simulink model "Deviation"  (R2021b)
settings: Solver=VariableStepAuto  StartTime=0.0  StopTime=100  RelTol=1e-3
undefined symbols (not defined in the file or in its folder): A, B, B_pseudoinverse, C, F, K
settings Model: Creator=Asus  LastModifiedBy=Asus

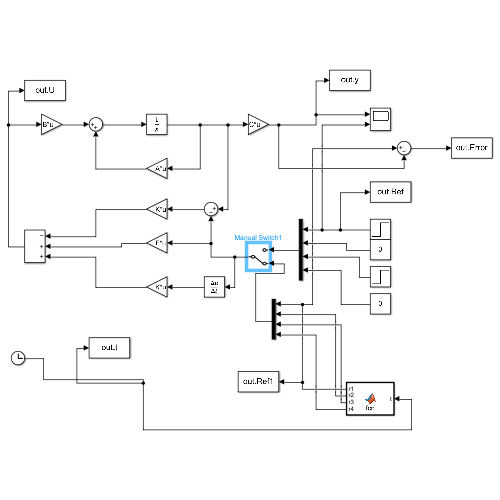
[thumbnail: Simulink's stored preview of the top-level diagram]
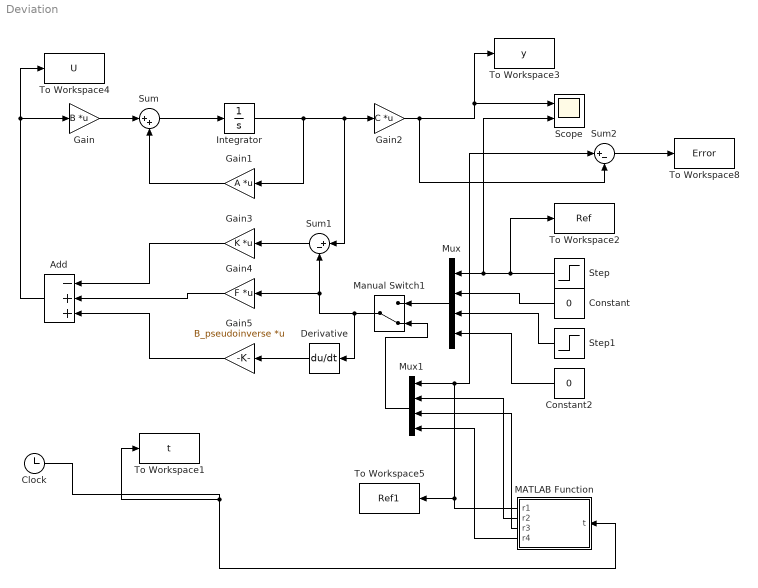
== system Deviation ==
  Add : Sum  Inputs=-++
  Clock : Clock
  Constant : Constant  Value=0
  Constant2 : Constant  Value=0
  Derivative : Derivative
  Gain : Gain  Gain=B  Multiplication=Matrix(K*u)
  Gain1 : Gain  Gain=A  Multiplication=Matrix(K*u)
  Gain2 : Gain  Gain=C  Multiplication=Matrix(K*u)
  Gain3 : Gain  Gain=K  Multiplication=Matrix(K*u)
  Gain4 : Gain  Gain=F  Multiplication=Matrix(K*u)
  Gain5 : Gain  Gain=B_pseudoinverse  Multiplication=Matrix(K*u)
  Integrator : Integrator
  MATLAB Function : MATLAB Function  TreatAsAtomicUnit=on
  Manual Switch1 : ManualSwitch  CurrentSetting=0
  Mux : Mux
  Mux1 : Mux
  Scope : Scope  NumInputPorts=2
  Step : Step  After=10  SampleTime=0
  Step1 : Step  After=10  SampleTime=0
  Sum : Sum  Inputs=|++
  Sum1 : Sum  Inputs=|+-
  Sum2 : Sum  Inputs=|+-
  To Workspace1 : ToWorkspace  VariableName=t  SaveFormat=Timeseries  SampleTime=-1
  To Workspace2 : ToWorkspace  VariableName=Ref  SaveFormat=Timeseries  SampleTime=-1
  To Workspace3 : ToWorkspace  VariableName=y  SaveFormat=Timeseries  SampleTime=-1
  To Workspace4 : ToWorkspace  VariableName=U  SaveFormat=Timeseries  SampleTime=-1
  To Workspace5 : ToWorkspace  VariableName=Ref1  SaveFormat=Timeseries  SampleTime=-1
  To Workspace8 : ToWorkspace  VariableName=Error  SaveFormat=Timeseries  SampleTime=-1
  wires:
  Gain/1 -> Sum/1
  Sum/1 -> Integrator/1
  Gain3/1 -> Add/1
  Gain4/1 -> Add/2
  Gain5/1 -> Add/3
  Add/1 -> To Workspace4/1, Gain/1
  Integrator/1 -> Gain1/1, Sum1/1, Gain2/1
  Gain1/1 -> Sum/2
  Gain2/1 -> Sum2/2, To Workspace3/1, Scope/1
  Sum1/1 -> Gain3/1
  Derivative/1 -> Gain5/1
  Constant/1 -> Mux/2
  Step1/1 -> Mux/3
  Step/1 -> To Workspace2/1, Scope/2, Mux/1
  Constant2/1 -> Mux/4
  Clock/1 -> To Workspace1/1, MATLAB Function/1(t)
  Sum2/1 -> To Workspace8/1
  MATLAB Function/1(r1) -> To Workspace5/1, Sum2/1, Mux1/1
  MATLAB Function/2(r2) -> Mux1/2
  MATLAB Function/3(r3) -> Mux1/3
  MATLAB Function/4(r4) -> Mux1/4
  Mux/1 -> Manual Switch1/1
  Mux1/1 -> Manual Switch1/2
  Manual Switch1/1 -> Derivative/1, Gain4/1, Sum1/2

== matlab function Deviation/MATLAB Function ==
  data: t input; r1 output; r2 output; r3 output; r4 output
function [r1,r2,r3,r4]  = fcn(t)
r1 = sin(t);
r2 = cos(t);
r3 = sin(t);
r4 = cos(t);
